simulink model "Lorenza_2021b"  (R2021b)
settings: Solver=FixedStepAuto  StartTime=0.0  StopTime=25  FixedStep=0.001  RelTol=1e-3
settings Model: Creator=Tymon  LastModifiedBy=tymon

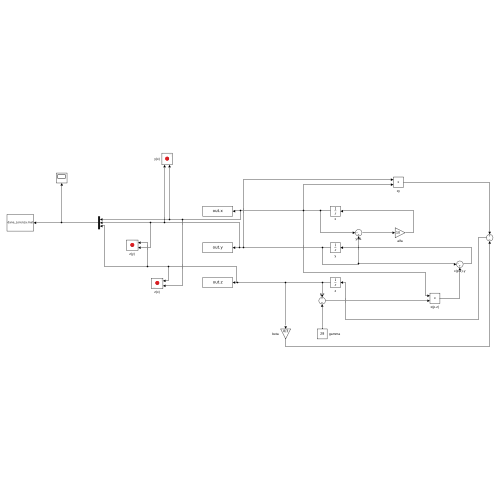
[thumbnail: Simulink's stored preview of the top-level diagram]
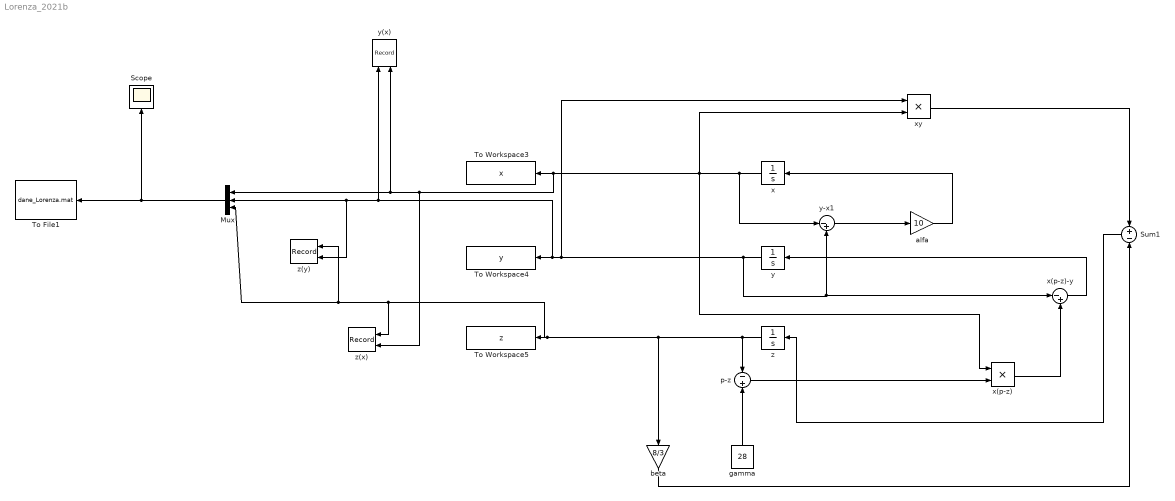
== system Lorenza_2021b ==
  Mux : Mux  Inputs=3
  Scope : Scope
  Sum1 : Sum  Inputs=+-
  To File1 : ToFile  Filename=dane_Lorenza.mat  MatrixName=dane_Lorenza
  To Workspace3 : ToWorkspace  VariableName=x  SampleTime=-1
  To Workspace4 : ToWorkspace  VariableName=y  SampleTime=-1
  To Workspace5 : ToWorkspace  VariableName=z  SampleTime=-1
  alfa : Gain  Gain=10
  beta : Gain  Gain=8/3
  gamma : Constant  Value=28
  p-z : Sum  Inputs=-+
  x : Integrator  InitialCondition=1
  x(p-z) : Product
  x(p-z)-y : Sum  Inputs=|-+
  xy : Product
  y : Integrator  InitialCondition=1
  y(x) : Record  FileSettingsInternal="{\"entries\":[{\"content\":{\"excelSettings\":{\"content\":{},\"type\":\"Streamout.ExcelSettings\"}},\"type\":\"Streamout.FileSettingStorage\",\"uuid\":\"927f2628-a168-4b2f-888a-0bcf40694843\"}],\"packageUris\":[\"http://schema.mathworks.com/mf0/streamout_blocks/R2020a\"],\"version\":\"1.0\"}"  Layout=[1 1]  SignalsInternal="{\"entries\":[{\"content\":{\"signals\":[{\"content\":{\"blockPath\":[\"Lorenza_2021b/y(x)\"],\"channel\":[],\"dimensions\":[1],\"domain\":\"Lorenza_2021b/y(x)\",\"lineColor\":\"#b746ff\",\"plots\":[1],\"port\":1,\"sid\":[],\"signalID\":49,\"signalName\":\"y\"},\"type\":\"RecordBlkView.Signal\",\"uuid\":\"6b18b6db-33fe-4578-babd-5da748080f56\"},{\"content\":{\"blockPath\":[\"Lorenza_2021b/y(x)\"],\"channel\":[],\"dimensions\":[1],\"domain\":\"Lorenza_2021b/y(x)\",\"lineColor\":\"#b746ff\",\"plots\":[1],\"port\":2,\"sid\":[],\"signalID\":52,\"signalName\":\"x\"},\"type\":\"RecordBlkView.Signal\",\"uuid\":\"8577aff2-7825-4e82-95e9-bfb54924e671\"}]},\"type\":\"RecordBlkView.InputSignals\",\"uuid\":\"9fa52f2b-58e6-459b-901c-e1a2955c1553\"}],\"packageUris\":[\"http://schema.mathworks.com/mf0/streamout_blocks/R2020a\"],\"version\":\"1.0\"}"  VisualizationBindings="{\"xyplotplugin\":{\"info\":[{\"series\":[{\"bindingParametersList\":[{\"parameter\":\"Y-Axis\",\"signalID\":52,\"signalName\":\"x\"},{\"parameter\":\"X-Axis\",\"signalID\":49,\"signalName\":\"y\"}],\"seriesID\":20467}],\"subplotID\":1}]}}"  CompatibilityTag=XY
  y-x1 : Sum  Inputs=|-+
  z : Integrator  InitialCondition=1
  z(x) : Record  FileSettingsInternal="{\"entries\":[{\"content\":{\"excelSettings\":{\"content\":{},\"type\":\"Streamout.ExcelSettings\"}},\"type\":\"Streamout.FileSettingStorage\",\"uuid\":\"407f7174-1f42-4e6c-ac8c-99c3da51c8e5\"}],\"packageUris\":[\"http://schema.mathworks.com/mf0/streamout_blocks/R2020a\"],\"version\":\"1.0\"}"  Layout=[1 1]  SignalsInternal="{\"entries\":[{\"content\":{\"signals\":[{\"content\":{\"blockPath\":[\"Lorenza_2021b/z(x)\"],\"channel\":[],\"dimensions\":[1],\"domain\":\"Lorenza_2021b/z(x)\",\"lineColor\":\"#ff13a6\",\"plots\":[1],\"port\":1,\"sid\":[],\"signalID\":41,\"signalName\":\"z\"},\"type\":\"RecordBlkView.Signal\",\"uuid\":\"aeebff78-708f-4922-82b4-71713c69dc83\"},{\"content\":{\"blockPath\":[\"Lorenza_2021b/z(x)\"],\"channel\":[],\"dimensions\":[1],\"domain\":\"Lorenza_2021b/z(x)\",\"lineColor\":\"#fe330a\",\"plots\":[1],\"port\":2,\"sid\":[],\"signalID\":44,\"signalName\":\"x\"},\"type\":\"RecordBlkView.Signal\",\"uuid\":\"f7f31d1c-d64d-45eb-96fc-a35ebd551108\"}]},\"type\":\"RecordBlkView.InputSignals\",\"uuid\":\"cf55bf82-86f9-4c8f-a4e5-64f88299321a\"}],\"packageUris\":[\"http://schema.mathworks.com/mf0/streamout_blocks/R2020a\"],\"version\":\"1.0\"}"  VisualizationBindings="{\"xyplotplugin\":{\"info\":[{\"series\":[{\"bindingParametersList\":[{\"parameter\":\"Y-Axis\",\"signalID\":41,\"signalName\":\"z\"},{\"parameter\":\"X-Axis\",\"signalID\":44,\"signalName\":\"x\"}],\"seriesID\":22268}],\"subplotID\":1}]}}"  CompatibilityTag=XY
  z(y) : Record  FileSettingsInternal="{\"entries\":[{\"content\":{\"excelSettings\":{\"content\":{},\"type\":\"Streamout.ExcelSettings\"}},\"type\":\"Streamout.FileSettingStorage\",\"uuid\":\"268a56d3-78e9-4ded-b37f-d0f5a6ed243e\"}],\"packageUris\":[\"http://schema.mathworks.com/mf0/streamout_blocks/R2020a\"],\"version\":\"1.0\"}"  Layout=[1 1]  SignalsInternal="{\"entries\":[{\"content\":{\"signals\":[{\"content\":{\"blockPath\":[\"Lorenza_2021b/z(y)\"],\"channel\":[],\"dimensions\":[1],\"domain\":\"Lorenza_2021b/z(y)\",\"lineColor\":\"#22b573\",\"plots\":[1],\"port\":1,\"sid\":[],\"signalID\":33,\"signalName\":\"z\"},\"type\":\"RecordBlkView.Signal\",\"uuid\":\"5a44c897-e7b3-472d-8e90-2dac52640ac7\"},{\"content\":{\"blockPath\":[\"Lorenza_2021b/z(y)\"],\"channel\":[],\"dimensions\":[1],\"domain\":\"Lorenza_2021b/z(y)\",\"lineColor\":\"#0072bd\",\"plots\":[1],\"port\":2,\"sid\":[],\"signalID\":36,\"signalName\":\"y\"},\"type\":\"RecordBlkView.Signal\",\"uuid\":\"8516fca5-764d-49b8-a7b4-9911105d6089\"}]},\"type\":\"RecordBlkView.InputSignals\",\"uuid\":\"ffaadcda-16eb-4a87-8003-f33a97a89890\"}],\"packageUris\":[\"http://schema.mathworks.com/mf0/streamout_blocks/R2020a\"],\"version\":\"1.0\"}"  VisualizationBindings="{\"xyplotplugin\":{\"info\":[{\"series\":[{\"bindingParametersList\":[{\"parameter\":\"Y-Axis\",\"signalID\":36,\"signalName\":\"y\"},{\"parameter\":\"X-Axis\",\"signalID\":33,\"signalName\":\"z\"}],\"seriesID\":46368}],\"subplotID\":1}]}}"  CompatibilityTag=XY
  wires:
  x/1 -> y-x1/1, xy/2, x(p-z)/1, z(x)/2, y(x)/2, Mux/1, To Workspace3/1
  y/1 -> xy/1, y(x)/1, z(y)/2, Mux/2, To Workspace4/1, y-x1/2, x(p-z)-y/1
  z/1 -> beta/1, z(x)/1, z(y)/1, Mux/3, To Workspace5/1, p-z/1
  y-x1/1 -> alfa/1
  alfa/1 -> x/1
  gamma/1 -> p-z/2
  p-z/1 -> x(p-z)/2
  x(p-z)/1 -> x(p-z)-y/2
  x(p-z)-y/1 -> y/1
  beta/1 -> Sum1/2
  xy/1 -> Sum1/1
  Sum1/1 -> z/1
  Mux/1 -> Scope/1, To File1/1
